simulink model "PrioritySignalSelector"  (R2025a)
settings: Solver=VariableStepAuto  StartTime=0.0  StopTime=10.0  RelTol=1e-3
settings Model: Creator=mahij  LastModifiedBy=mahij

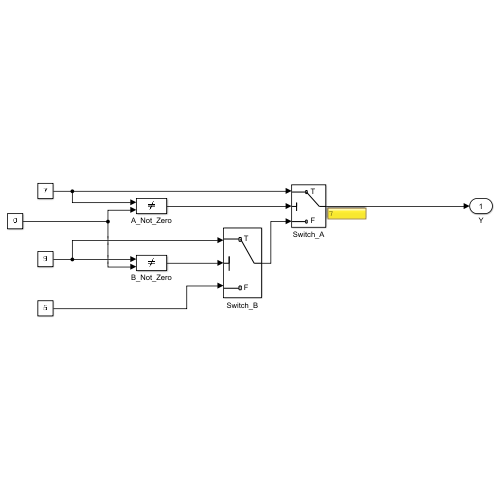
[thumbnail: Simulink's stored preview of the top-level diagram]
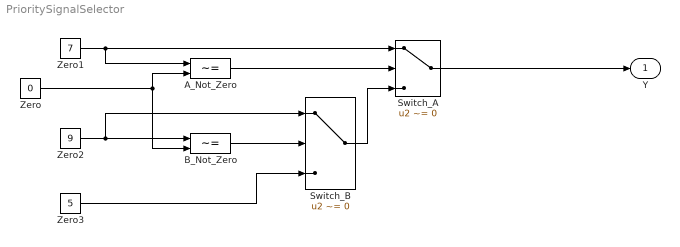
== system PrioritySignalSelector ==
  A_Not_Zero : RelationalOperator  Operator=~=  OutDataTypeStr=boolean  RndMeth=Simplest  InputSameDT=off
  B_Not_Zero : RelationalOperator  Operator=~=  OutDataTypeStr=boolean  RndMeth=Simplest  InputSameDT=off
  Switch_A : Switch  Criteria=u2 ~= 0  SaturateOnIntegerOverflow=off  InputSameDT=off
  Switch_B : Switch  Criteria=u2 ~= 0  SaturateOnIntegerOverflow=off  InputSameDT=off
  Zero : Constant  Value=0
  Zero1 : Constant  Value=7
  Zero2 : Constant  Value=9
  Zero3 : Constant  Value=5
  Y : Outport
  wires:
  Zero/1 -> A_Not_Zero/2, B_Not_Zero/2
  Zero1/1 -> A_Not_Zero/1, Switch_A/1
  Zero2/1 -> Switch_B/1, B_Not_Zero/1
  A_Not_Zero/1 -> Switch_A/2
  B_Not_Zero/1 -> Switch_B/2
  Zero3/1 -> Switch_B/3
  Switch_B/1 -> Switch_A/3
  Switch_A/1 -> Y/1
